simulink model "Subsystem"  (R2020b)
settings: Solver=VariableStepAuto  StartTime=0.0  StopTime=10.0  RelTol=1e-3
settings Model: Creator=Dell  LastModifiedBy=Dell
settings DataIOCC: SaveOutput=off  SaveTime=off

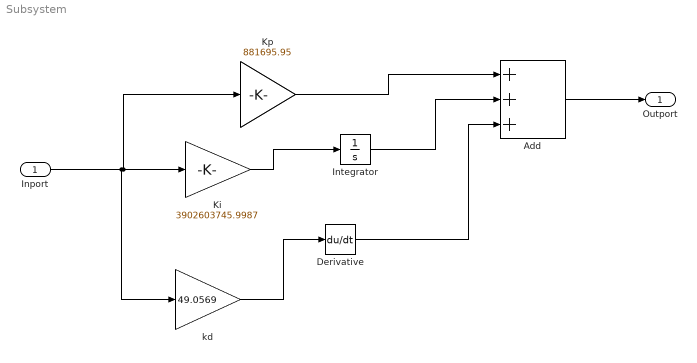
== system Subsystem ==
  Inport : Inport  OutDataTypeStr=double  PortDimensions=1  SampleTime=0
  Add : Sum  Inputs=+++
  Derivative : Derivative
  Integrator : Integrator
  Ki : Gain  Gain=3902603745.9987
  Kp : Gain  Gain=881695.95
  kd : Gain  Gain=49.0569
  Outport : Outport  OutDataTypeStr=double  PortDimensions=1  SampleTime=0
  wires:
  Kp/1 -> Add/1
  Derivative/1 -> Add/3
  Ki/1 -> Integrator/1
  Inport/1 -> Kp/1, Ki/1, kd/1
  kd/1 -> Derivative/1
  Add/1 -> Outport/1
  Integrator/1 -> Add/2
